simulink model "bh_1dof_CONFIRM_SIGN_CONVENTION"  (R2016b)
settings: Solver=ode15s  StartTime=0.0  StopTime=20  MaxStep=0.01  RelTol=1e-3  EnableMultiTasking=on
PreLoadFcn:
  | bh_script_1dof_params_CONFIRM_SIGN_CONVENTION
values from neighbouring files (symbols this model uses):
  c = 2*0.2*3    (= 1.2)    [bh_script_1dof_params_CONFIRM_SIGN_CONVENTION.m]
  xC0 = x0    (= 1)    [bh_script_1dof_params_CONFIRM_SIGN_CONVENTION.m]
  xDEF0 = xR0 - xC0    (= -1)    [bh_script_1dof_params_CONFIRM_SIGN_CONVENTION.m]
  xR0 = 0    [bh_script_1dof_params_CONFIRM_SIGN_CONVENTION.m]
libraries: fl_lib x10, nesl_utility x5
Description:
  | Copyright 2014 The MathWorks, Inc.
settings Model: Creator=smiller  LastModifiedBy=bhorton
settings DataIOCC: LimitDataPoints=on  SaveFormat=Array
settings OptimizationCC: LifeSpan=inf
settings DebuggingCC: UnderspecifiedInitializationDetection=Classic  MergeDetectMultiDrivingBlocksExec=none  SolverPrmCheckMsg=warning  AllowSymbolicDim=off  StateNameClashWarn=warning  SFUnexpectedBacktrackingDiag=warning  SFNoUnconditionalDefaultTransitionDiag=warning  SFExecutionAtInitializationDiag=none
settings HardwareCC: ProdBitPerPointer=32  ProdBitPerSizeT=32  ProdBitPerPtrDiffT=32  ProdLargestAtomicFloat=None  ProdIntDivRoundTo=Undefined  ProdEndianess=Unspecified  ProdWordSize=32  ProdHWDeviceType=32-bit Generic
settings ModelReferenceCC: PropagateSignalLabelsOutOfModel=off
settings GRTTargetCC: TargetLangStandard=C89/C90 (ANSI)  GeneratePreprocessorConditionals=Disable all
settings ConfigComp: CovMetricSettings=dw  CovHtmlReporting=on  CovSaveCumulativeToWorkspaceVar=on  CovSaveSingleToWorkspaceVar=on  CovExternalEMLEnable=off  CovSFcnEnable=off

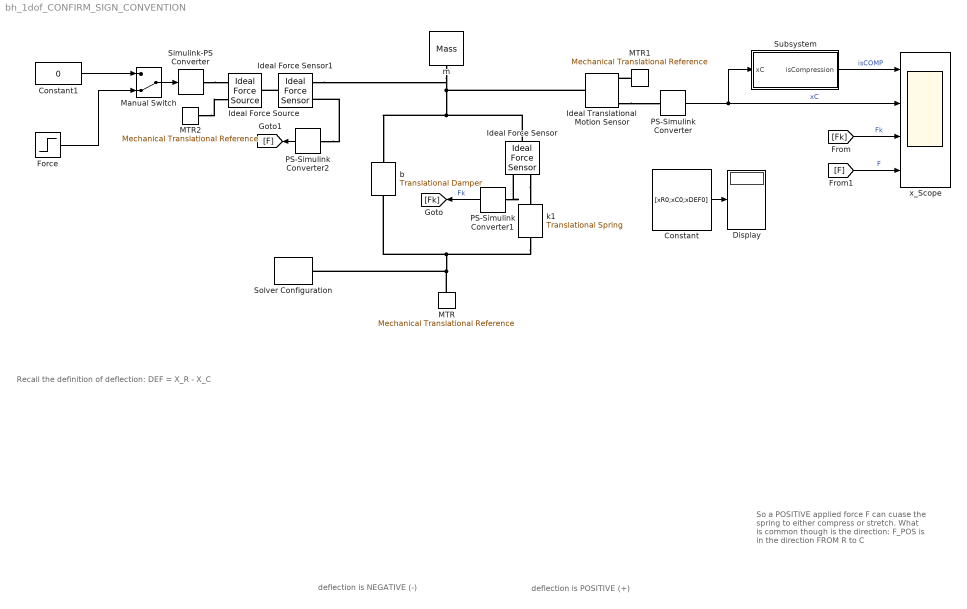
== system bh_1dof_CONFIRM_SIGN_CONVENTION ==
  note: So a POSITIVE applied force F
      | can cuase the spring to either compress
      | or stretch.
      |
      | What is common though is the direction:
      |
      | F_POS is in the direction FROM R to C
  note: Recall the definition of deflection:
      |
      |          DEF = X_R - X_C
  note: deflection is NEGATIVE (-)
  note: deflection is POSITIVE (+)
  Constant : Constant  Value=[xR0;xC0;xDEF0]  VectorParams1D=off
  Constant1 : Constant  Value=0
  Display : Display
  Force : Step  Time=15  After=9  SampleTime=0
      settings: AttributesFormatString=|
      | Time of step = %<Time>
      | Final value = %<After>
  Ideal Force Sensor : fl_lib/Mechanical/Mechanical Sensors/Ideal Force Sensor
  Ideal Force Sensor1 : fl_lib/Mechanical/Mechanical Sensors/Ideal Force Sensor
  Ideal Force Source : fl_lib/Mechanical/Mechanical Sources/Ideal Force Source
  Ideal Translational Motion Sensor : fl_lib/Mechanical/Mechanical Sensors/Ideal Translational Motion Sensor  offset=xC0 m
      settings: AttributesFormatString=offset = %<offset>
  MTR : fl_lib/Mechanical/Translational Elements/Mechanical Translational Reference
  MTR1 : fl_lib/Mechanical/Translational Elements/Mechanical Translational Reference
  MTR2 : fl_lib/Mechanical/Translational Elements/Mechanical Translational Reference
  Manual Switch : ManualSwitch  CurrentSetting=0
  PS-Simulink Converter : nesl_utility/PS-Simulink Converter  PhysicalDomain=network_engine_domain  SubClassName=ps_output  LeftPortType=input  RightPortType=output  PseudoPeriodic=off  Frequencies=[]  Unit=m  AffineConversion=off
  PS-Simulink Converter1 : nesl_utility/PS-Simulink Converter  PhysicalDomain=network_engine_domain  SubClassName=ps_output  LeftPortType=input  RightPortType=output  PseudoPeriodic=off  Frequencies=[]  Unit=N  AffineConversion=off
  PS-Simulink Converter2 : nesl_utility/PS-Simulink Converter  PhysicalDomain=network_engine_domain  SubClassName=ps_output  LeftPortType=input  RightPortType=output  PseudoPeriodic=off  Frequencies=[]  Unit=N  AffineConversion=off
  Simulink-PS Converter : nesl_utility/Simulink-PS Converter  PhysicalDomain=network_engine_domain  SubClassName=ps_input  LeftPortType=input  RightPortType=output  PseudoPeriodic=off  Frequencies=[]  NoiseDistribution=none  NoiseParameters=[]  Unit=N  AffineConversion=off  InputFiltering=off  SimscapeFilterOrder=1  InputFilterTimeConstant=.001  UdotUserProvided=0
  Solver Configuration : nesl_utility/Solver Configuration  PhysicalDomain=network_engine_domain  SubClassName=solver  LeftPortType=input  RightPortType=generic  Accelerate=off  Tones=[]  Harmonics=[]  SimulateNoise=off  Profile=off  UseLocalSampling=off  EnableSwitchedLinearOptims=on  FrequencyDomain=off  UseCCode=off  RelTol=0.001  AbsTol=1e-06  MinStep=1e-09  ToWorkspace=off  RevertToSquareIcSolve=off  NumHomotopyIterations=100  PhasorMode=off  PhasorModeNumHarmonics=1  OverrideAbsTol=off  DoDC=off  ResidualTolerance=1e-9  UseLocalSolver=off  LocalSolverChoice=NE_BACKWARD_EULER_ADVANCER  LocalSolverSampleTime=.001  DoFixedCost=off  MaxNonlinIter=12  MaxModeIter=2  LinearAlgebra=Sparse  DelaysMemoryBudget=1024  AutomaticFiltering=on  FilteringTimeConstant=0.001
  Subsystem : Subsystem
  b : fl_lib/Mechanical/Translational Elements/Translational Damper  D=c N/(m/s)  v_specify=off  v_priority=None  v=0 m/s  f_specify=off  f_priority=None  f=0 N
  k1 : fl_lib/Mechanical/Translational Elements/Translational Spring  spr_rate=k N/m  v_specify=off  v_priority=High  v=xdot_0 m/s  f_specify=off  f_priority=None  f=0 N  x_specify=on  x_priority=High  x=xDEF0 m
      settings: AttributesFormatString=|
      | DEF_X = %<x>
      | K = %<spr_rate>
  m : fl_lib/Mechanical/Translational Elements/Mass  mass=m kg  v_specify=on  v_priority=None  v=xdot_0 m/s  f_specify=off  f_priority=None  f=0 N
      settings: AttributesFormatString=V0 = %<v>
  x_Scope : Scope  NumInputPorts=4
  wires:
  Force/1 -> Manual Switch/2
  PS-Simulink Converter/1 -> Subsystem/1(xC), x_Scope/2  "xC"
  Constant/1 -> Display/1
  Constant1/1 -> Manual Switch/1
  Manual Switch/1 -> Simulink-PS Converter/1
  PS-Simulink Converter1/1 -> [Fk]  "Fk"
  [Fk] -> x_Scope/3  "Fk"
  Subsystem/1(isCompression) -> x_Scope/1  "isCOMP"
  [F] -> x_Scope/4  "F"
  PS-Simulink Converter2/1 -> [F]
  connections:
  MTR2/LConn1 -- Ideal Force Source/RConn2
  MTR1/LConn1 -- Ideal Translational Motion Sensor/RConn1
  Ideal Translational Motion Sensor/RConn3 -- PS-Simulink Converter/LConn1
  Simulink-PS Converter/RConn1 -- Ideal Force Source/RConn1
  k1/LConn1 -- b/LConn1 -- MTR/LConn1 -- Solver Configuration/RConn1
  Ideal Force Sensor/RConn1 -- k1/RConn1
  PS-Simulink Converter1/LConn1 -- Ideal Force Sensor/RConn2
  Ideal Translational Motion Sensor/LConn1 -- Ideal Force Sensor1/RConn1 -- m/LConn1 -- b/RConn1 -- Ideal Force Sensor/LConn1
  Ideal Force Sensor1/LConn1 -- Ideal Force Source/LConn1
  PS-Simulink Converter2/LConn1 -- Ideal Force Sensor1/RConn2

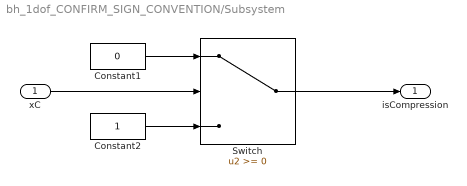
== system bh_1dof_CONFIRM_SIGN_CONVENTION/Subsystem ==
  xC : Inport
  Constant1 : Constant  Value=0
  Constant2 : Constant
  Switch : Switch
  isCompression : Outport
  wires:
  xC/1 -> Switch/2
  Constant1/1 -> Switch/1
  Constant2/1 -> Switch/3
  Switch/1 -> isCompression/1
